simulink model "BugE_v0_40_MAS_loads_opt"  (R2015b)
settings: Solver=FixedStepDiscrete  StartTime=0.0  StopTime=1370  FixedStep=sample_time  RelTol=1e-3
values from neighbouring files (symbols this model uses):
  AB_diode_dV = 0.9    [main_sync.m]
  air_density = 1.225    [main_sync.m]
  bus_ac_Pmax_abs = 240    [main_sync.m]
  bus_charger_Pmax = 1000    [main_sync.m]
  bus_load_Pmax_abs = 260    [main_sync.m]
  capInitVolt = capVmax*sqrt(capInitSoC)    [main_sync.m]
  cyc_kph = [cyc_kph(:,1), cyc_kph(:,2)*speed_max_limit/speed_max]    [main_sync.m]
  cyc_repeat = 1    [main_sync.m]
  ess1_init_soc = 1    [main_sync.m]
  ess1_soh = 1    [main_sync.m]
  ess2_init_soc = 1    [main_sync.m]
  ess2_soh = 1    [main_sync.m]
  ess3_init_soc = 1    [main_sync.m]
  ess3_soh = 1    [main_sync.m]
  ess4_init_soc = 1    [main_sync.m]
  ess4_soh = 1    [main_sync.m]
  ess5_init_soc = 1    [main_sync.m]
  ess5_soh = 1    [main_sync.m]
  gear_ratio = 6    [main_sync.m]
  JADE_on = 0    [main_sync.m]
  loadpower = rawcsv(:,2)    [main_sync.m]
  loadtime = rawcsv(:,1)    [main_sync.m]
  lockSOCs = 0    [main_sync.m]
  max_brk_torque = 300    [main_sync.m]
  no_wheels = 3    [main_sync.m]
  perform_sample_time = 3*60    (= 180)    [main_sync.m]
  period2 = max(loadtime)    [main_sync.m]
  PV_Pmax = 100    [main_sync.m]
  sample_time = 0.01    [main_sync.m]
  startup_seq_step_delay = 0.2    [main_sync.m]
  stop_option = 0    [main_sync.m]
  use_drive_cycle = 1    [main_sync.m]
  use_real_subs_loads = 1    [main_sync.m]
  vbus_max = 25    [main_sync.m]
  vbus_min = 17    [main_sync.m]
  vbus_safety_threshold = 2    [main_sync.m]
  vbus_threshold = 20    [main_sync.m]
  veh_CD = 0.35    [main_sync.m]
  veh_FA = 1.543    [main_sync.m]
  veh_gravity = 9.81*veh_mass    (= 1863.9)    [main_sync.m]
  veh_mass = 190    [main_sync.m]
  wh_1st_rrc = 0.02    [main_sync.m]
  wh_bearing_frc = 0.0015    [main_sync.m]
  wh_inertia = 0.0556    [main_sync.m]
  wh_radius = 0.508/2    (= 0.254)    [main_sync.m]
undefined symbols (not defined in the file or in its folder): capC, capR, cyc_acc, cyc_avg_time_samples, cyc_brk, cyc_grade, cyc_key, DCM_eff_factor_for_Vin, DCM_eff_for_Iout, DCM_Iout, DCM_Iout_max, DCM_Pin_noload, DCM_Pout_max, DCM_Vin, DCM_Vout, DiscIntNeverNeededParam, ess2_coulombic_eff, ess2_Ineg_max_SOC, ess2_Ineg_max_temp, ess2_Ipos_max_SOC, ess2_Ipos_max_temp, ess2_max_ah_cap, ess2_max_volts, ess2_min_volts, ess2_module_parallel, ess2_module_series, ess2_r_dis, ess2_soc, ess2_SOC_for_Ilimit, ess2_temp_for_Ilimit, ess2_temp_max, ess2_tmp, ess2_voc, ess3_coulombic_eff, ess3_max_ah_cap, ess3_module_parallel, ess3_module_series, ess3_r_dis, ess3_soc, ess3_tmp, ess3_voc, ess_coulombic_eff, ess_Ineg_max_SOC, ess_Ineg_max_temp, ess_Ipos_max_SOC, ess_Ipos_max_temp, ess_max_ah_cap, ess_max_volts, ess_min_volts, ess_module_parallel, ess_module_series, ess_nominal_volts, ess_r_dis, ess_soc, ess_SOC_for_Ilimit, ess_temp_for_Ilimit, ess_temp_max, ess_tmp, ess_voc, MC_eff1 ... (+18)
libraries: simulink x142, dspstat3 x2, commfilt2 x1, simulink_extras x1
(part 5 of 7)

== system BugE_v0_40_MAS_loads_opt/Master Controller/DCDC Calculators/FE // CHG Class Voltage => Power Droop ==
  Vbus_min : Inport
  Vbus_max : Inport  Port=2
  Vbus : Inport  Port=3
  Pmax_spec : Inport  Port=4
  50ms moving avg : DiscreteFir  Coefficients=ones(1,0.05*(1/sample_time))/(0.05*(1/sample_time))  SampleTime=sample_time
  >=0 : Saturate  UpperLimit=inf  LowerLimit=0
  Constant6 : Constant  SampleTime=sample_time
  Divide : Product  Inputs=*/
  Product : Product
  Subtract1 : Sum  Inputs=+-
  Subtract2 : Sum  Inputs=++-
  Subtract3 : Sum  Inputs=+-
  Subtract4 : Sum  Inputs=+-
  Subtract5 : Sum  Inputs=-+
  "[0,1]" : Saturate  UpperLimit=1-eps  LowerLimit=0
  beta : Constant  Value=0.9  SampleTime=sample_time
  sqr : Math  Operator=square  SaturateOnIntegerOverflow=on
  vf : Product  Inputs=*/
  Pmax_lim : Outport
  wires:
  Product/1 -> >=0/1
  Divide/1 -> Subtract2/3
  beta/1 -> Subtract3/2
  Subtract3/1 -> sqr/1
  sqr/1 -> Subtract2/2, Divide/1
  Constant6/1 -> Subtract2/1, Subtract3/1, Subtract4/1
  vf/1 -> "[0,1]"/1
  Subtract4/1 -> Divide/2
  >=0/1 -> Pmax_lim/1
  Vbus/1 -> 50ms moving avg/1
  Vbus_min/1 -> Subtract5/1, Subtract1/2
  Vbus_max/1 -> Subtract5/2
  Subtract5/1 -> vf/2
  Subtract1/1 -> vf/1
  "[0,1]"/1 -> Subtract4/2
  Subtract2/1 -> Product/1
  Pmax_spec/1 -> Product/2
  50ms moving avg/1 -> Subtract1/1

== system BugE_v0_40_MAS_loads_opt/Master Controller/DCDC Calculators/LD Class Voltage => Power Droop ==
  Vbus_min : Inport
  Vbus_max : Inport  Port=2
  Vbus : Inport  Port=3
  Pmax_spec_abs : Inport  Port=4
  50ms moving avg : DiscreteFir  Commented=through  Coefficients=ones(1,0.05*(1/sample_time))/(0.05*(1/sample_time))  SampleTime=sample_time
  <=0 : Saturate  UpperLimit=0  LowerLimit=-inf
  Constant6 : Constant  SampleTime=sample_time
  Divide1 : Product  Inputs=*/
  Product : Product
  Scope : Scope  NumInputPorts=2
  Subtract : Sum  Inputs=--+
  Subtract1 : Sum  Inputs=+-
  Subtract2 : Sum  Inputs=+-
  Subtract5 : Sum  Inputs=-+
  "[0,1]" : Saturate  UpperLimit=1  LowerLimit=eps
  beta : Constant  Value=0.9  SampleTime=sample_time
  sqr : Math  Operator=square  SaturateOnIntegerOverflow=on
  vf : Product  Inputs=*/
  Pmax_lim (neg) : Outport
  wires:
  vf/1 -> Scope/1, "[0,1]"/1
  50ms moving avg/1 -> Subtract1/1
  Vbus_min/1 -> Subtract5/1, Subtract1/2
  Vbus_max/1 -> Subtract5/2
  Subtract5/1 -> vf/2
  Subtract1/1 -> vf/1
  Constant6/1 -> Subtract/1, Subtract2/1
  beta/1 -> Subtract2/2
  Divide1/1 -> Subtract/3
  Subtract2/1 -> sqr/1
  sqr/1 -> Subtract/2, Divide1/1
  "[0,1]"/1 -> Divide1/2
  <=0/1 -> Scope/2, Pmax_lim (neg)/1
  Subtract/1 -> Product/1
  Pmax_spec_abs/1 -> Product/2
  Product/1 -> <=0/1
  Vbus/1 -> 50ms moving avg/1

== system BugE_v0_40_MAS_loads_opt/Master Controller/DCDC Calculators/ones voltage cmd ==
  I : Inport
  2dbl : DataTypeConversion
  Bias : Bias  Bias=1
  Gain : Gain  Gain=0
  O : Outport
  wires:
  Gain/1 -> Bias/1
  I/1 -> 2dbl/1
  2dbl/1 -> Gain/1
  Bias/1 -> O/1

== system BugE_v0_40_MAS_loads_opt/Master Controller/DCDC Calculators/zeros power cmd ==
  I : Inport
  2dbl : DataTypeConversion
  Gain : Gain  Gain=0
  O : Outport
  wires:
  Gain/1 -> O/1
  I/1 -> 2dbl/1
  2dbl/1 -> Gain/1

== system BugE_v0_40_MAS_loads_opt/Master Controller/DCDC Calculators/zeros power cmd1 ==
  I : Inport
  2dbl : DataTypeConversion
  Gain : Gain  Gain=0
  O : Outport
  wires:
  Gain/1 -> O/1
  I/1 -> 2dbl/1
  2dbl/1 -> Gain/1

== system BugE_v0_40_MAS_loads_opt/Master Controller/Motor Controller/MB Class Current => Throttle Droop ==
  I : Inport
  Imax : Inport  Port=2
  Constant6 : Constant  SampleTime=sample_time
  Divide : Product  Inputs=*/
  If : Product  Inputs=*/
  Rate Limiter 0-full in 1s : RateLimiter  FallingSlewLimit=-1/sample_time  SampleTimeMode=inherited  LinearizeAsGain=off
  Subtract2 : Sum  Inputs=++-
  Subtract3 : Sum  Inputs=+-
  Subtract4 : Sum  Inputs=+-
  "[0, 1]" : Saturate  UpperLimit=1-eps  LowerLimit=0
  "[0,1-eps]" : Saturate  UpperLimit=1-eps  LowerLimit=0
  beta : Constant  Value=0.85  SampleTime=sample_time
  moving average 200ms : DiscreteFir  Coefficients=ones(1,20)/20  SampleTime=sample_time
  sqr : Math  Operator=square  SaturateOnIntegerOverflow=on
  thr_max_lim : Outport
  wires:
  Subtract2/1 -> "[0, 1]"/1
  Divide/1 -> Subtract2/3
  beta/1 -> Subtract3/2
  Subtract3/1 -> sqr/1
  sqr/1 -> Subtract2/2, Divide/1
  Constant6/1 -> Subtract2/1, Subtract3/1, Subtract4/1
  Subtract4/1 -> Divide/2
  "[0,1-eps]"/1 -> Subtract4/2
  Imax/1 -> If/2
  If/1 -> "[0,1-eps]"/1
  "[0, 1]"/1 -> Rate Limiter 0-full in 1s/1
  Rate Limiter 0-full in 1s/1 -> moving average 200ms/1
  moving average 200ms/1 -> thr_max_lim/1
  I/1 -> If/1

== system BugE_v0_40_MAS_loads_opt/Master Controller/Operating Mode Controller/Accessories (State 2) ==
  note: Disable for MB modules
      | where the DCDC is ok but
      | the battery is not usable;
      |
      | Enable for everything usable
  devices_ON bus : Inport
  Enable : EnablePort  StatesWhenEnabling=reset
  Bus Creator1 : BusCreator  Inputs=10
  Bus Creator2 : BusCreator  Inputs=5
  Bus Selector : BusSelector  OutputSignals=MBDCDC_on,MB_on,SBDCDC_on,SB_on,FEDCDC_on,FE_on,CHGDCDC_on,CHG_on,LDDCDC_on,LD_on
  Constant : Constant  OutDataTypeStr=boolean  SampleTime=sample_time
  and{5..9} (5 alike) : Logic  AllPortsSameDT=off  OutDataTypeStr=boolean
  not{,1..4} (5 alike) : Logic  Operator=NOT  AllPortsSameDT=off  OutDataTypeStr=boolean
  pass : Subsystem
  pass5 : Subsystem
  pass6 : Subsystem
  pass7 : Subsystem
  RLYs_and_12V bus : Outport  OutputWhenDisabled=reset  InitialOutput=0
  droop_bus : Outport  Port=2  OutputWhenDisabled=reset  InitialOutput=0
  wires:
  Constant/1 -> Bus Creator2/5  "RLY_DRV_DSBL"
  Bus Creator1/1 -> droop_bus/1
  devices_ON bus/1 -> Bus Selector/1
  and5/1 -> pass6/1(I), not/1, Bus Creator1/1  "MB_droop_EN"
  and7/1 -> not2/1, Bus Creator1/3  "FE_droop_EN"
  and8/1 -> not3/1, Bus Creator1/4  "CHG_droop_EN"
  and6/1 -> pass7/1(I), not1/1, Bus Creator1/2  "SB_droop_EN"
  and9/1 -> not4/1, Bus Creator1/5  "LD_droop_EN"
  Bus Selector/1 -> and5/1  "<MBDCDC_on>"
  Bus Selector/10 -> and9/2  "<LD_on>"
  Bus Selector/9 -> and9/1  "<LDDCDC_on>"
  Bus Selector/8 -> and8/2  "<CHG_on>"
  Bus Selector/7 -> and8/1  "<CHGDCDC_on>"
  Bus Selector/6 -> and7/2  "<FE_on>"
  Bus Selector/5 -> and7/1  "<FEDCDC_on>"
  Bus Selector/4 -> and6/2  "<SB_on>"
  Bus Selector/3 -> and6/1  "<SBDCDC_on>"
  Bus Selector/2 -> and5/2  "<MB_on>"
  not/1 -> pass5/1(I), Bus Creator1/6  "MB_droop_DSBL"
  not1/1 -> pass/1(I), Bus Creator1/7  "SB_droop_DSBL"
  not2/1 -> Bus Creator1/8  "FE_droop_DSBL"
  not3/1 -> Bus Creator1/9  "CHG_droop_DSBL"
  not4/1 -> Bus Creator1/10  "LD_droop_DSBL"
  Bus Creator2/1 -> RLYs_and_12V bus/1
  pass/1(O) -> Bus Creator2/1  "RLY_SB_DSBL"
  pass5/1(O) -> Bus Creator2/2  "RLY_MB_DSBL"
  pass6/1(O) -> Bus Creator2/3  "RLY_MB_EN"
  pass7/1(O) -> Bus Creator2/4  "RLY_SB_EN"

== system BugE_v0_40_MAS_loads_opt/Master Controller/Operating Mode Controller/Driving (State 3) ==
  note: Everything usable including
      | MB modules where the
      | DCDC is ok but the battery
      | is not usable (fail-mode)
  devices_ON bus : Inport
  Enable : EnablePort  StatesWhenEnabling=reset
  Bus Creator1 : BusCreator  Inputs=10
  Bus Creator2 : BusCreator  Inputs=5
  Bus Selector : BusSelector  OutputSignals=MBDCDC_on,MB_on,SBDCDC_on,SB_on,FEDCDC_on,FE_on,CHGDCDC_on,CHG_on,LDDCDC_on,LD_on
  Constant : Constant  OutDataTypeStr=boolean  SampleTime=sample_time
  and{6..9} (4 alike) : Logic  AllPortsSameDT=off  OutDataTypeStr=boolean
  not{,1..5} (6 alike) : Logic  Operator=NOT  AllPortsSameDT=off  OutDataTypeStr=boolean
  pass{2..5} (4 alike) : Logic  Operator=NOT  AllPortsSameDT=off  OutDataTypeStr=boolean
  through{2..5} (4 alike) : Logic  Operator=NOT  AllPortsSameDT=off  OutDataTypeStr=boolean
  RLYs_and_12V bus : Outport  OutputWhenDisabled=reset  InitialOutput=0
  droop_bus : Outport  Port=2  OutputWhenDisabled=reset  InitialOutput=0
  wires:
  Constant/1 -> Bus Creator2/5  "RLY_DRV_EN"
  Bus Creator1/1 -> droop_bus/1
  devices_ON bus/1 -> Bus Selector/1
  through5/1 -> Bus Creator1/1  "MB_droop_EN"
  and7/1 -> not2/1, Bus Creator1/3  "FE_droop_EN"
  and8/1 -> not3/1, Bus Creator1/4  "CHG_droop_EN"
  and6/1 -> pass4/1, not1/1, Bus Creator1/2  "SB_droop_EN"
  and9/1 -> not4/1, Bus Creator1/5  "LD_droop_EN"
  Bus Selector/1 -> not/1, pass5/1  "<MBDCDC_on>"
  Bus Selector/10 -> and9/2  "<LD_on>"
  Bus Selector/9 -> and9/1  "<LDDCDC_on>"
  Bus Selector/8 -> and8/2  "<CHG_on>"
  Bus Selector/7 -> and8/1  "<CHGDCDC_on>"
  Bus Selector/6 -> and7/2  "<FE_on>"
  Bus Selector/5 -> and7/1  "<FEDCDC_on>"
  Bus Selector/4 -> and6/2  "<SB_on>"
  Bus Selector/3 -> and6/1  "<SBDCDC_on>"
  Bus Selector/2 -> pass3/1, not5/1  "<MB_on>"
  not/1 -> Bus Creator1/6  "MB_droop_DSBL"
  not1/1 -> Bus Creator1/7, pass2/1  "SB_droop_DSBL"
  not2/1 -> Bus Creator1/8  "FE_droop_DSBL"
  not3/1 -> Bus Creator1/9  "CHG_droop_DSBL"
  not4/1 -> Bus Creator1/10  "LD_droop_DSBL"
  Bus Creator2/1 -> RLYs_and_12V bus/1
  pass2/1 -> through2/1
  through2/1 -> Bus Creator2/1  "RLY_SB_DSBL"
  not5/1 -> Bus Creator2/2  "RLY_MB_DSBL"
  pass3/1 -> through3/1
  through3/1 -> Bus Creator2/3  "RLY_MB_EN"
  pass4/1 -> through4/1
  through4/1 -> Bus Creator2/4  "RLY_SB_EN"
  pass5/1 -> through5/1

== system BugE_v0_40_MAS_loads_opt/Master Controller/Operating Mode Controller/Standby (State 0) ==
  devices_ON bus : Inport
  Enable : EnablePort  StatesWhenEnabling=reset
  Bus Creator : BusCreator  Inputs=5
  Bus Creator1 : BusCreator  Inputs=6
  Bus Creator2 : BusCreator  Inputs=5
  Bus Selector : BusSelector  OutputSignals=MBDCDC_on,SBDCDC_on,FEDCDC_on,CHGDCDC_on,LDDCDC_on
  dbl2bool{,1..15} (16 alike) : DataTypeConversion  OutDataTypeStr=boolean
  disable everything : Constant  OutDataTypeStr=double  SampleTime=sample_time
  ones : Subsystem
  ones1 : Subsystem
  ones2 : Subsystem
  ones3 : Subsystem
  ones4 : Subsystem
  RLYs_and_12V bus : Outport  OutputWhenDisabled=reset  InitialOutput=0
  module_PWR bus : Outport  Port=2  OutputWhenDisabled=reset  InitialOutput=0
  droop_bus : Outport  Port=3  OutputWhenDisabled=reset  InitialOutput=0
  wires:
  Bus Selector/1 -> ones/1(I)  "<MBDCDC_on>"
  Bus Selector/2 -> ones1/1(I)  "<SBDCDC_on>"
  Bus Selector/3 -> ones2/1(I)  "<FEDCDC_on>"
  Bus Selector/4 -> ones3/1(I)  "<CHGDCDC_on>"
  Bus Selector/5 -> ones4/1(I)  "<LDDCDC_on>"
  dbl2bool2/1 -> Bus Creator/1  "MB_droop_DSBL"
  dbl2bool1/1 -> Bus Creator/2  "SB_droop_DSBL"
  dbl2bool/1 -> Bus Creator/3  "FE_droop_DSBL"
  dbl2bool3/1 -> Bus Creator/5  "LD_droop_DSBL"
  dbl2bool4/1 -> Bus Creator/4  "CHG_droop_DSBL"
  Bus Creator/1 -> droop_bus/1
  devices_ON bus/1 -> Bus Selector/1  "detected and not turned off internally"
  Bus Creator2/1 -> module_PWR bus/1
  dbl2bool8/1 -> Bus Creator2/5  "LD_PWR_DSBL"
  dbl2bool9/1 -> Bus Creator2/4  "CHG_PWR_DSBL"
  dbl2bool5/1 -> Bus Creator2/3  "FE_PWR_DSBL"
  dbl2bool6/1 -> Bus Creator2/2  "SB_MOD_PWR_DSBL"
  dbl2bool7/1 -> Bus Creator2/1  "MB_MOD_PWR_DSBL"
  dbl2bool10/1 -> Bus Creator1/6  "RLY_SB_DSBL"
  dbl2bool11/1 -> Bus Creator1/5  "RLY_MB_DSBL"
  dbl2bool14/1 -> Bus Creator1/1  "DDC_DSBL"
  dbl2bool13/1 -> Bus Creator1/2  "RLY_EDLC_DSBL"
  dbl2bool12/1 -> Bus Creator1/3  "RLY_AUX_DSBL"
  dbl2bool15/1 -> Bus Creator1/4  "RLY_DRV_DSBL"
  disable everything/1 -> dbl2bool15/1, dbl2bool12/1, dbl2bool13/1, dbl2bool14/1
  Bus Creator1/1 -> RLYs_and_12V bus/1
  ones/1(O) -> dbl2bool7/1, dbl2bool10/1, dbl2bool2/1
  ones1/1(O) -> dbl2bool11/1, dbl2bool6/1, dbl2bool1/1
  ones2/1(O) -> dbl2bool5/1, dbl2bool/1
  ones3/1(O) -> dbl2bool9/1, dbl2bool4/1
  ones4/1(O) -> dbl2bool8/1, dbl2bool3/1

== system BugE_v0_40_MAS_loads_opt/Master Controller/Operating Mode Controller/Startup sequence (State 1) ==
  note: STEP 1.
      | 	enable module power
      | 	for All energy sources
      | STEP 2.
      | 	close EDLC relays (DOT)
      | STEP 3.
      | 	close BMU batt relays via CAN
      | STEP 4.
      | 	enable Droop control for
      | 	everything but loads
      |
      | When the bus is ready (charged)...
      |
      | STEP 5.
      | 	enable DDC, loads, Droop
      | 	for everything
      | STEP 6.
      | 	disable power for all modules
      | 	not being detected, and
      | 	set startup ready flag
  note: No loads or MB modules
      | where the DCDC is ok but
      | the battery is not usable
  note: No MB modules where
      | the DCDC is ok but
      | the battery is not usable
  devices_ON bus : Inport
  bus ready : Inport  Port=2
  Enable : EnablePort  StatesWhenEnabling=reset
  Bus Creator1 : BusCreator  Inputs=5
  Bus Creator2 : BusCreator  Inputs=10
  Bus Selector2 : BusSelector  OutputSignals=LDDCDC_on,MBDCDC_on,SBDCDC_on,FEDCDC_on,CHGDCDC_on,MB_on,SB_on,FE_on,CHG_on,LD_on
  Switch : Switch  Criteria=u2 > Threshold
  Switch1 : Switch  Criteria=u2 > Threshold
  and{,1..11} (12 alike) : Logic  AllPortsSameDT=off  OutDataTypeStr=boolean
  choose_droop_activations : Subsystem  TreatAsAtomicUnit=on
  choose_droop_activations1 : Subsystem  TreatAsAtomicUnit=on
  nor{,1..4} (5 alike) : Logic  Operator=NOR  AllPortsSameDT=off  OutDataTypeStr=boolean
  ones : Subsystem
  ones1 : Subsystem
  ones2 : Subsystem
  ones3 : Subsystem
  ones4 : Subsystem
  pass : Subsystem
  pass1 : Subsystem
  start : Constant  OutDataTypeStr=boolean  SampleTime=sample_time
  startup_seq_step_delay w/ latch : Subsystem
  zeros : Subsystem
  RLYs_and_12V bus : Outport  OutputWhenDisabled=reset  InitialOutput=0
  droop_bus : Outport  Port=2  OutputWhenDisabled=reset  InitialOutput=0
  SUR : Outport  Port=3  OutputWhenDisabled=reset  InitialOutput=0
  module_PWR bus : Outport  Port=4  OutputWhenDisabled=reset  InitialOutput=0
  wires:
  startup_seq_step_delay w/ latch/2(delayed 2x) -> and2/1, and/1
  startup_seq_step_delay w/ latch/3(delayed 3x) -> Switch1/2, choose_droop_activations/Enable
  bus ready/1 -> startup_seq_step_delay w/ latch/2(bus ready)
  Switch/1 -> droop_bus/1
  choose_droop_activations1/1(droop_EN bus) -> Switch/1
  and1/1 -> Bus Creator2/6  "MB_MOD_PWR_EN"
  and4/1 -> Bus Creator2/7  "SB_MOD_PWR_EN"
  ones1/1(O) -> and3/1
  Switch1/1 -> Switch/3
  and5/1 -> Bus Creator2/10  "LD_PWR_EN"
  and6/1 -> Bus Creator2/9  "CHG_PWR_EN"
  and3/1 -> Bus Creator2/8  "FE_PWR_EN"
  and2/1 -> Bus Creator1/3  "RLY_SB_EN"
  and/1 -> Bus Creator1/2  "RLY_MB_EN"
  pass/1(O) -> Bus Creator1/4  "DDC_EN"
  pass1/1(O) -> Bus Creator1/5  "RLY_AUX_EN"
  Bus Creator1/1 -> RLYs_and_12V bus/1
  start/1 -> and6/2, and1/2, and4/2, and3/2, startup_seq_step_delay w/ latch/1(sigin)
  ones2/1(O) -> and4/1
  ones3/1(O) -> and6/1
  Bus Selector2/7 -> nor1/2, ones2/1(I)  "<SB_on>"
  Bus Selector2/9 -> nor3/2, ones3/1(I)  "<CHG_on>"
  startup_seq_step_delay w/ latch/1(delayed) -> Bus Creator1/1  "RLY_EDLC_EN"
  Bus Selector2/8 -> nor2/2, ones1/1(I), and2/2  "<FE_on>"
  Bus Selector2/6 -> ones/1(I), nor/2, and/2  "<MB_on>"
  ones/1(O) -> and1/1
  startup_seq_step_delay w/ latch/4(delayed 4x & BR) -> and5/2, choose_droop_activations1/Enable, Switch/2, pass1/1(I), pass/1(I)
  choose_droop_activations/1(droop_EN bus) -> Switch1/1
  zeros/1(O) -> Switch1/3
  devices_ON bus/1 -> choose_droop_activations/1(devices_ON bus), choose_droop_activations1/1(devices_ON bus), zeros/1(I), Bus Selector2/1
  Bus Selector2/2 -> nor/1  "<MBDCDC_on>"
  Bus Selector2/10 -> nor4/2, ones4/1(I)  "<LD_on>"
  Bus Selector2/1 -> nor4/1  "<LDDCDC_on>"
  Bus Selector2/5 -> nor3/1  "<CHGDCDC_on>"
  Bus Selector2/4 -> nor2/1  "<FEDCDC_on>"
  Bus Selector2/3 -> nor1/1  "<SBDCDC_on>"
  and7/1 -> Bus Creator2/2  "MB_PWR_DSBL"
  and8/1 -> Bus Creator2/3  "SB_PWR_DSBL"
  and9/1 -> Bus Creator2/4  "FE_PWR_DSBL"
  and10/1 -> Bus Creator2/5  "CHG_PWR_DSBL"
  and11/1 -> Bus Creator2/1  "LD_PWR_DSBL"
  Bus Creator2/1 -> module_PWR bus/1
  nor2/1 -> and9/2
  nor1/1 -> and8/2
  nor/1 -> and7/2
  nor3/1 -> and10/2
  nor4/1 -> and11/1
  startup_seq_step_delay w/ latch/5((d4x & BR) delayed 2x) -> and10/1, and9/1, and8/1, and7/1, and11/2, SUR/1
  ones4/1(O) -> and5/1

== system BugE_v0_40_MAS_loads_opt/Master Controller/Operating Mode Controller/State machine 0 std, 1 startup, 2 acc, 3 drv, 4 fault ==
  ACC : Inport
  IGON : Inport  Port=2
  RFD (ready for driving) : Inport  Port=3
  SUR (startup ready) : Inport  Port=4
  ESTOP (user triggered e-stop) : Inport  Port=5
  0 => 1 : Subsystem  TreatAsAtomicUnit=on
  1 => 2 : Subsystem  TreatAsAtomicUnit=on
  2 => 3 : Subsystem  TreatAsAtomicUnit=on
  3 => 2 : Subsystem  TreatAsAtomicUnit=on
  ==0 : simulink/Logic and Bit Operations/Compare To Constant  relop===  const=0  OutDataTypeStr=boolean
  ==1 : simulink/Logic and Bit Operations/Compare To Constant  relop===  const=1  OutDataTypeStr=boolean
  ==2 : simulink/Logic and Bit Operations/Compare To Constant  relop===  const=2  OutDataTypeStr=boolean
  ==3 : simulink/Logic and Bit Operations/Compare To Constant  relop===  const=3  OutDataTypeStr=boolean
  All => 0 : Subsystem  TreatAsAtomicUnit=on
  If : If  NumInputs=6  IfExpression=((~u2) & (~u3)) | u6  ElseIfExpressions="(u1==0) & u2,  (u1==1) & u2 & u4,  (u1==2) & u3 & u5,  (u1==3) & ((~u3)|(~u5))"
  New state Default 0 : Merge  Inputs=6  InitialOutput=0
  Old state 1 : UnitDelay  SampleTime=sample_time
  bool2dbl {2..6} (5 alike) : DataTypeConversion  OutDataTypeStr=double
  maintain : Subsystem  TreatAsAtomicUnit=on
  pass10 : Subsystem
  pass2 : Subsystem
  pass3 : Subsystem
  pass4 : Subsystem
  pass5 : Subsystem
  state : Outport
  enable_standby : Outport  Port=2
  enable_startup : Outport  Port=3
  enable_accessories : Outport  Port=4
  enable_driving : Outport  Port=5
  wires:
  pass5/1(O) -> bool2dbl 5/1  "ems_SM_RFD"
  If/1 -> All => 0/Action
  If/2 -> 0 => 1/Action
  If/3 -> 1 => 2/Action
  If/4 -> 2 => 3/Action
  If/5 -> 3 => 2/Action
  If/6 -> maintain/Action
  3 => 2/1(new) -> New state Default 0/5
  maintain/1(new) -> New state Default 0/6
  pass2/1(O) -> bool2dbl 2/1  "ems_SM_ACC"
  pass3/1(O) -> bool2dbl 3/1  "ems_SM_IGON"
  ==1/1 -> enable_startup/1
  ==2/1 -> enable_accessories/1
  ==3/1 -> enable_driving/1
  ==0/1 -> enable_standby/1
  pass4/1(O) -> bool2dbl 4/1  "ems_SM_SUR"
  bool2dbl 3/1 -> If/3
  bool2dbl 2/1 -> If/2
  bool2dbl 5/1 -> If/5
  bool2dbl 4/1 -> If/4
  bool2dbl 6/1 -> If/6
  New state Default 0/1 -> ==3/1, ==2/1, ==1/1, Old state 1/1, state/1, ==0/1  "ems_SM_state"
  Old state 1/1 -> If/1, maintain/1(prev)
  All => 0/1(new) -> New state Default 0/1
  2 => 3/1(new) -> New state Default 0/4
  1 => 2/1(new) -> New state Default 0/3
  0 => 1/1(new) -> New state Default 0/2
  pass10/1(O) -> bool2dbl 6/1  "ems_SM_ESTOP"
  ACC/1 -> pass2/1(I)
  IGON/1 -> pass3/1(I)
  SUR (startup ready)/1 -> pass4/1(I)
  RFD (ready for driving)/1 -> pass5/1(I)
  ESTOP (user triggered e-stop)/1 -> pass10/1(I)

== system BugE_v0_40_MAS_loads_opt/Master Controller/Operating Mode Controller/bus charged & within limits ==
  < vbus_max + (...) : RelationalOperator  Operator=<  OutDataTypeStr=boolean
  >= vbus_threshold : simulink/Logic and Bit Operations/Compare To Constant  relop=>=  const=vbus_threshold  OutDataTypeStr=boolean
  Add : Sum
  Logical Operator : Logic  AllPortsSameDT=off  OutDataTypeStr=boolean
  vbus_max : Constant  Value=vbus_max  SampleTime=sample_time
  vbus_safety_threshold : Constant  Value=vbus_safety_threshold  SampleTime=sample_time
  bus_ready : Outport
  wires:
  >= vbus_threshold/1 -> Logical Operator/1
  [Vcap_reading] -> < vbus_max + (...)/1, >= vbus_threshold/1
  Add/1 -> < vbus_max + (...)/2
  vbus_max/1 -> Add/1
  vbus_safety_threshold/1 -> Add/2
  Logical Operator/1 -> bus_ready/1
  < vbus_max + (...)/1 -> Logical Operator/2

== system BugE_v0_40_MAS_loads_opt/Master Controller/Operating Mode Controller/ready for driving ==
  Bus Selector : BusSelector  OutputSignals=MBDCDC_on,MB_on
  From11 : From  Commented=on  GotoTag=CHGDCDC_detected  TagVisibility=global
  From12 : From  Commented=on  GotoTag=CHG_detected  TagVisibility=global
  a charger connected : Logic  Operator=OR  Inputs=1  AllPortsSameDT=off  OutDataTypeStr=boolean
  able to power motor : Logic  Inputs=1  AllPortsSameDT=off  OutDataTypeStr=boolean
  and : Logic  AllPortsSameDT=off  OutDataTypeStr=boolean
  no charger connected : Logic  Operator=NOT  Inputs=1  AllPortsSameDT=off  OutDataTypeStr=boolean
  or : Logic  Operator=OR  AllPortsSameDT=off  OutDataTypeStr=boolean
  ready : Logic  AllPortsSameDT=off  OutDataTypeStr=boolean
  RFD : Outport
  wires:
  and/1 -> a charger connected/1
  ready/1 -> RFD/1
  or/1 -> able to power motor/1
  no charger connected/1 -> ready/1
  able to power motor/1 -> ready/2
  From12/1 -> and/2
  From11/1 -> and/1
  [devices_ON_bus] -> Bus Selector/1
  Bus Selector/1 -> or/1  "<MBDCDC_on>"
  Bus Selector/2 -> or/2  "<MB_on>"
  a charger connected/1 -> no charger connected/1

== system BugE_v0_40_MAS_loads_opt/Master Controller/Operating Mode Controller/start-up ready ==
  Compare To Zero : simulink/Logic and Bit Operations/Compare To Zero  relop===  OutDataTypeStr=boolean
  S-R Flip-Flop : simulink_extras/Flip Flops/S-R Flip-Flop  initial_condition=0
  Terminator : Terminator
  Unit Delay : UnitDelay  SampleTime=sample_time
  Unit Delay1 : UnitDelay  SampleTime=sample_time
  SUR : Outport
  wires:
  [SM_SUR_flag] -> Unit Delay/1
  [state] -> Unit Delay1/1
  Unit Delay/1 -> S-R Flip-Flop/1
  Compare To Zero/1 -> S-R Flip-Flop/2
  Unit Delay1/1 -> Compare To Zero/1
  S-R Flip-Flop/1 -> SUR/1
  S-R Flip-Flop/2 -> Terminator/1

== system BugE_v0_40_MAS_loads_opt/Master Controller/Secondary Objectives/MB SOC balancing ==
  enable : Inport
  "Balancing type: 1: none, 2: P>0, 3: P<0" : Subsystem
  Bus Selector : BusSelector  OutputSignals=MB_droop
  MB balancing through load distribution : Subsystem
  Mux1 : Mux  Inputs=2
  Mux2 : Mux  Inputs=2
  Scope : Scope
  and : Logic  AllPortsSameDT=off  OutDataTypeStr=boolean
  MB slope adj : Outport
  wires:
  MB balancing through load distribution/1(MB slope adj) -> MB slope adj/1
  enable/1 -> "Balancing type: 1: none, 2: P>0, 3: P<0"/1(enable)
  Mux1/1 -> "Balancing type: 1: none, 2: P>0, 3: P<0"/2(DCDC Iout (bus side))
  [active_droop_bus] -> Bus Selector/1
  [RLY_MB] -> and/2
  "Balancing type: 1: none, 2: P>0, 3: P<0"/1(type) -> MB balancing through load distribution/1(distribution type), Scope/1
  Mux2/1 -> MB balancing through load distribution/3(MB SOCs)
  and/1 -> "Balancing type: 1: none, 2: P>0, 3: P<0"/3(enabled MODs), MB balancing through load distribution/2(MOD's EN)
  Bus Selector/1 -> and/1  "<MB_droop>"
  [Iout_MB1_DCDC_reading] -> Mux1/1
  [Iout_MB2_DCDC_reading] -> Mux1/2
  [SOC_MB1_received] -> Mux2/1
  [SOC_MB2_received] -> Mux2/2

== system BugE_v0_40_MAS_loads_opt/Master Controller/Secondary Objectives/Motor MBDCDC boost ==
  enable : Inport
  Bus Selector : BusSelector  OutputSignals=MB_droop
  Product : Product
  Saturation : Saturate  UpperLimit=0  LowerLimit=vbus_min-vbus_max
  Switch1 : Switch  Criteria=u2 > Threshold
  "[0.05, inf)" : DeadZone  LowerValue=-inf  UpperValue=0.05  SaturateOnIntegerOverflow=on
  boost off : Logic  Operator=NOT  AllPortsSameDT=off  OutDataTypeStr=boolean
  d Imotor / d t : simulink/Discrete/Discrete Derivative  gainval=1.0  ICPrevScaledInput=0.0  InputProcessing=Inherited  OutMin=[]  OutMax=[]  OutDataType=fixdt(1, 16)  OutScaling=2^-10  DoSatur=off
  moving average 50ms : DiscreteFir  Coefficients=ones(1,5)/5  SampleTime=sample_time
  normalize 1 / Imax : Gain  Gain=1/mc_max_crrnt
  ones : Subsystem
  shift gain [d_V0/ (d_I/d_t)] : Gain  Gain=-25
  some MB DCDCs are off : Logic  Operator=NAND  Inputs=1  AllPortsSameDT=off  OutDataTypeStr=boolean
  use boost : Logic  Operator=NOR  AllPortsSameDT=off  OutDataTypeStr=boolean
  zero : Constant  Value=0  SampleTime=sample_time
  MB V0 adj : Outport
  wires:
  shift gain [d_V0/ (d_I/d_t)]/1 -> Saturation/1
  moving average 50ms/1 -> normalize 1 / Imax/1
  enable/1 -> boost off/1
  boost off/1 -> use boost/2
  use boost/1 -> Switch1/2
  some MB DCDCs are off/1 -> use boost/1
  Product/1 -> Switch1/1
  zero/1 -> Switch1/3
  ones/1(O) -> Product/2
  normalize 1 / Imax/1 -> d Imotor / d t/1
  [Drive_current_reading] -> moving average 50ms/1
  Switch1/1 -> MB V0 adj/1
  d Imotor / d t/1 -> "[0.05, inf)"/1
  "[0.05, inf)"/1 -> shift gain [d_V0/ (d_I/d_t)]/1
  Saturation/1 -> Product/1
  [active_droop_bus] -> Bus Selector/1
  Bus Selector/1 -> ones/1(I), some MB DCDCs are off/1  "<MB_droop>"

== system BugE_v0_40_MAS_loads_opt/Master Controller/Secondary Objectives/Source prioritization ==
  enable : Inport
  Bias : Bias  Bias=1
  Bus Selector1 : BusSelector  OutputSignals=CHG_droop,MB_droop,SB_droop
  Gain : Gain  Gain=-1
  Gain1 : Gain  Gain=-2
  Product : Product
  Product1 : Product
  and1 : Logic  AllPortsSameDT=off  OutDataTypeStr=boolean
  and2 : Logic  AllPortsSameDT=off  OutDataTypeStr=boolean
  bool2dbl : DataTypeConversion  OutDataTypeStr=double
  bool2dbl1 : DataTypeConversion  OutDataTypeStr=double
  bool2dbl2 : DataTypeConversion  OutDataTypeStr=double
  charging : Logic  Operator=OR  Inputs=1  AllPortsSameDT=off  OutDataTypeStr=boolean
  SB slope adj : Outport
  MB V0 adj : Outport  Port=2
  SB V0 adj : Outport  Port=3
  wires:
  Bus Selector1/3 -> and1/1  "<SB_droop>"
  Bus Selector1/1 -> charging/1  "<CHG_droop>"
  charging/1 -> bool2dbl/1
  [active_droop_bus] -> Bus Selector1/1
  bool2dbl/1 -> Product1/1, Product/1
  Product/1 -> Gain1/1
  Product1/1 -> Gain/1
  Bias/1 -> SB slope adj/1
  and2/1 -> bool2dbl1/1
  bool2dbl2/1 -> Bias/1, Product1/2
  bool2dbl1/1 -> Product/2
  enable/1 -> and2/2, and1/2
  and1/1 -> bool2dbl2/1
  Bus Selector1/2 -> and2/1  "<MB_droop>"
  Gain1/1 -> MB V0 adj/1
  Gain/1 -> SB V0 adj/1

== system BugE_v0_40_MAS_loads_opt/Master Controller/Signal Buffer/(0 device OFF // 1 ON)1 ==
  EN : Inport
  DSBL : Inport  Port=2
  2dbl : DataTypeConversion  OutDataTypeStr=double
  2dbl1 : DataTypeConversion  OutDataTypeStr=double
  Detect Increase : simulink/Logic and Bit Operations/Detect Increase  vinit=0.0  InputProcessing=Inherited  OutDataTypeStr=boolean
  Detect Increase1 : simulink/Logic and Bit Operations/Detect Increase  vinit=0.0  InputProcessing=Inherited  OutDataTypeStr=boolean
  OR : Sum
  Switch : Switch  Criteria=u2 > Threshold
  Switch1 : Switch  Criteria=u2 > Threshold
  Unit Delay : UnitDelay  SampleTime=sample_time
  disable : Constant  Value=0  OutDataTypeStr=boolean  SampleTime=sample_time
  enable : Constant  OutDataTypeStr=boolean  SampleTime=sample_time
  state : Outport
  wires:
  EN/1 -> Detect Increase/1
  Detect Increase1/1 -> 2dbl1/1
  Switch/1 -> state/1, Unit Delay/1
  DSBL/1 -> Detect Increase1/1
  OR/1 -> Switch/2
  Detect Increase/1 -> 2dbl/1
  Unit Delay/1 -> Switch/3
  disable/1 -> Switch1/1
  enable/1 -> Switch1/3
  Switch1/1 -> Switch/1
  2dbl1/1 -> Switch1/2, OR/2
  2dbl/1 -> OR/1

== system BugE_v0_40_MAS_loads_opt/Master Controller/Signal Buffer/(0 device OFF // 1 ON)10 ==
  EN : Inport
  DSBL : Inport  Port=2
  2dbl : DataTypeConversion  OutDataTypeStr=double
  2dbl1 : DataTypeConversion  OutDataTypeStr=double
  Detect Increase : simulink/Logic and Bit Operations/Detect Increase  vinit=0.0  InputProcessing=Inherited  OutDataTypeStr=boolean
  Detect Increase1 : simulink/Logic and Bit Operations/Detect Increase  vinit=0.0  InputProcessing=Inherited  OutDataTypeStr=boolean
  OR : Sum
  Switch : Switch  Criteria=u2 > Threshold
  Switch1 : Switch  Criteria=u2 > Threshold
  Unit Delay : UnitDelay  SampleTime=sample_time
  disable : Constant  Value=0  OutDataTypeStr=boolean  SampleTime=sample_time
  enable : Constant  OutDataTypeStr=boolean  SampleTime=sample_time
  state : Outport
  wires:
  EN/1 -> Detect Increase/1
  Detect Increase1/1 -> 2dbl1/1
  Switch/1 -> state/1, Unit Delay/1
  DSBL/1 -> Detect Increase1/1
  OR/1 -> Switch/2
  Detect Increase/1 -> 2dbl/1
  Unit Delay/1 -> Switch/3
  disable/1 -> Switch1/1
  enable/1 -> Switch1/3
  Switch1/1 -> Switch/1
  2dbl1/1 -> Switch1/2, OR/2
  2dbl/1 -> OR/1

== system BugE_v0_40_MAS_loads_opt/Master Controller/Signal Buffer/(0 device OFF // 1 ON)11 ==
  EN : Inport
  DSBL : Inport  Port=2
  2dbl : DataTypeConversion  OutDataTypeStr=double
  2dbl1 : DataTypeConversion  OutDataTypeStr=double
  Detect Increase : simulink/Logic and Bit Operations/Detect Increase  vinit=0.0  InputProcessing=Inherited  OutDataTypeStr=boolean
  Detect Increase1 : simulink/Logic and Bit Operations/Detect Increase  vinit=0.0  InputProcessing=Inherited  OutDataTypeStr=boolean
  OR : Sum
  Switch : Switch  Criteria=u2 > Threshold
  Switch1 : Switch  Criteria=u2 > Threshold
  Unit Delay : UnitDelay  SampleTime=sample_time
  disable : Constant  Value=0  OutDataTypeStr=boolean  SampleTime=sample_time
  enable : Constant  OutDataTypeStr=boolean  SampleTime=sample_time
  state : Outport
  wires:
  EN/1 -> Detect Increase/1
  Detect Increase1/1 -> 2dbl1/1
  Switch/1 -> state/1, Unit Delay/1
  DSBL/1 -> Detect Increase1/1
  OR/1 -> Switch/2
  Detect Increase/1 -> 2dbl/1
  Unit Delay/1 -> Switch/3
  disable/1 -> Switch1/1
  enable/1 -> Switch1/3
  Switch1/1 -> Switch/1
  2dbl1/1 -> Switch1/2, OR/2
  2dbl/1 -> OR/1

== system BugE_v0_40_MAS_loads_opt/Master Controller/Signal Buffer/(0 device OFF // 1 ON)12 ==
  EN : Inport
  DSBL : Inport  Port=2
  2dbl : DataTypeConversion  OutDataTypeStr=double
  2dbl1 : DataTypeConversion  OutDataTypeStr=double
  Detect Increase : simulink/Logic and Bit Operations/Detect Increase  vinit=0.0  InputProcessing=Inherited  OutDataTypeStr=boolean
  Detect Increase1 : simulink/Logic and Bit Operations/Detect Increase  vinit=0.0  InputProcessing=Inherited  OutDataTypeStr=boolean
  OR : Sum
  Switch : Switch  Criteria=u2 > Threshold
  Switch1 : Switch  Criteria=u2 > Threshold
  Unit Delay : UnitDelay  SampleTime=sample_time
  disable : Constant  Value=0  OutDataTypeStr=boolean  SampleTime=sample_time
  enable : Constant  OutDataTypeStr=boolean  SampleTime=sample_time
  state : Outport
  wires:
  EN/1 -> Detect Increase/1
  Detect Increase1/1 -> 2dbl1/1
  Switch/1 -> state/1, Unit Delay/1
  DSBL/1 -> Detect Increase1/1
  OR/1 -> Switch/2
  Detect Increase/1 -> 2dbl/1
  Unit Delay/1 -> Switch/3
  disable/1 -> Switch1/1
  enable/1 -> Switch1/3
  Switch1/1 -> Switch/1
  2dbl1/1 -> Switch1/2, OR/2
  2dbl/1 -> OR/1

== system BugE_v0_40_MAS_loads_opt/Master Controller/Signal Buffer/(0 device OFF // 1 ON)13 ==
  EN : Inport
  DSBL : Inport  Port=2
  2dbl : DataTypeConversion  OutDataTypeStr=double
  2dbl1 : DataTypeConversion  OutDataTypeStr=double
  Detect Increase : simulink/Logic and Bit Operations/Detect Increase  vinit=0.0  InputProcessing=Inherited  OutDataTypeStr=boolean
  Detect Increase1 : simulink/Logic and Bit Operations/Detect Increase  vinit=0.0  InputProcessing=Inherited  OutDataTypeStr=boolean
  OR : Sum
  Switch : Switch  Criteria=u2 > Threshold
  Switch1 : Switch  Criteria=u2 > Threshold
  Unit Delay : UnitDelay  SampleTime=sample_time
  disable : Constant  Value=0  OutDataTypeStr=boolean  SampleTime=sample_time
  enable : Constant  OutDataTypeStr=boolean  SampleTime=sample_time
  state : Outport
  wires:
  EN/1 -> Detect Increase/1
  Detect Increase1/1 -> 2dbl1/1
  Switch/1 -> state/1, Unit Delay/1
  DSBL/1 -> Detect Increase1/1
  OR/1 -> Switch/2
  Detect Increase/1 -> 2dbl/1
  Unit Delay/1 -> Switch/3
  disable/1 -> Switch1/1
  enable/1 -> Switch1/3
  Switch1/1 -> Switch/1
  2dbl1/1 -> Switch1/2, OR/2
  2dbl/1 -> OR/1

== system BugE_v0_40_MAS_loads_opt/Master Controller/Signal Buffer/(0 device OFF // 1 ON)14 ==
  EN : Inport
  DSBL : Inport  Port=2
  2dbl : DataTypeConversion  OutDataTypeStr=double
  2dbl1 : DataTypeConversion  OutDataTypeStr=double
  Detect Increase : simulink/Logic and Bit Operations/Detect Increase  vinit=0.0  InputProcessing=Inherited  OutDataTypeStr=boolean
  Detect Increase1 : simulink/Logic and Bit Operations/Detect Increase  vinit=0.0  InputProcessing=Inherited  OutDataTypeStr=boolean
  OR : Sum
  Switch : Switch  Criteria=u2 > Threshold
  Switch1 : Switch  Criteria=u2 > Threshold
  Unit Delay : UnitDelay  SampleTime=sample_time
  disable : Constant  Value=0  OutDataTypeStr=boolean  SampleTime=sample_time
  enable : Constant  OutDataTypeStr=boolean  SampleTime=sample_time
  state : Outport
  wires:
  EN/1 -> Detect Increase/1
  Detect Increase1/1 -> 2dbl1/1
  Switch/1 -> state/1, Unit Delay/1
  DSBL/1 -> Detect Increase1/1
  OR/1 -> Switch/2
  Detect Increase/1 -> 2dbl/1
  Unit Delay/1 -> Switch/3
  disable/1 -> Switch1/1
  enable/1 -> Switch1/3
  Switch1/1 -> Switch/1
  2dbl1/1 -> Switch1/2, OR/2
  2dbl/1 -> OR/1

== system BugE_v0_40_MAS_loads_opt/Master Controller/Signal Buffer/(0 device OFF // 1 ON)15 ==
  EN : Inport
  DSBL : Inport  Port=2
  2dbl : DataTypeConversion  OutDataTypeStr=double
  2dbl1 : DataTypeConversion  OutDataTypeStr=double
  Detect Increase : simulink/Logic and Bit Operations/Detect Increase  vinit=0.0  InputProcessing=Inherited  OutDataTypeStr=boolean
  Detect Increase1 : simulink/Logic and Bit Operations/Detect Increase  vinit=0.0  InputProcessing=Inherited  OutDataTypeStr=boolean
  OR : Sum
  Switch : Switch  Criteria=u2 > Threshold
  Switch1 : Switch  Criteria=u2 > Threshold
  Unit Delay : UnitDelay  SampleTime=sample_time
  disable : Constant  Value=0  OutDataTypeStr=boolean  SampleTime=sample_time
  enable : Constant  OutDataTypeStr=boolean  SampleTime=sample_time
  state : Outport
  wires:
  EN/1 -> Detect Increase/1
  Detect Increase1/1 -> 2dbl1/1
  Switch/1 -> state/1, Unit Delay/1
  DSBL/1 -> Detect Increase1/1
  OR/1 -> Switch/2
  Detect Increase/1 -> 2dbl/1
  Unit Delay/1 -> Switch/3
  disable/1 -> Switch1/1
  enable/1 -> Switch1/3
  Switch1/1 -> Switch/1
  2dbl1/1 -> Switch1/2, OR/2
  2dbl/1 -> OR/1

== system BugE_v0_40_MAS_loads_opt/Master Controller/Signal Buffer/(0 device OFF // 1 ON)16 ==
  EN : Inport
  DSBL : Inport  Port=2
  2dbl : DataTypeConversion  OutDataTypeStr=double
  2dbl1 : DataTypeConversion  OutDataTypeStr=double
  Detect Increase : simulink/Logic and Bit Operations/Detect Increase  vinit=0.0  InputProcessing=Inherited  OutDataTypeStr=boolean
  Detect Increase1 : simulink/Logic and Bit Operations/Detect Increase  vinit=0.0  InputProcessing=Inherited  OutDataTypeStr=boolean
  OR : Sum
  Switch : Switch  Criteria=u2 > Threshold
  Switch1 : Switch  Criteria=u2 > Threshold
  Unit Delay : UnitDelay  SampleTime=sample_time
  disable : Constant  Value=0  OutDataTypeStr=boolean  SampleTime=sample_time
  enable : Constant  OutDataTypeStr=boolean  SampleTime=sample_time
  state : Outport
  wires:
  EN/1 -> Detect Increase/1
  Detect Increase1/1 -> 2dbl1/1
  Switch/1 -> state/1, Unit Delay/1
  DSBL/1 -> Detect Increase1/1
  OR/1 -> Switch/2
  Detect Increase/1 -> 2dbl/1
  Unit Delay/1 -> Switch/3
  disable/1 -> Switch1/1
  enable/1 -> Switch1/3
  Switch1/1 -> Switch/1
  2dbl1/1 -> Switch1/2, OR/2
  2dbl/1 -> OR/1

== system BugE_v0_40_MAS_loads_opt/Master Controller/Signal Buffer/(0 device OFF // 1 ON)2 ==
  EN : Inport
  DSBL : Inport  Port=2
  2dbl : DataTypeConversion  OutDataTypeStr=double
  2dbl1 : DataTypeConversion  OutDataTypeStr=double
  Detect Increase : simulink/Logic and Bit Operations/Detect Increase  vinit=0.0  InputProcessing=Inherited  OutDataTypeStr=boolean
  Detect Increase1 : simulink/Logic and Bit Operations/Detect Increase  vinit=0.0  InputProcessing=Inherited  OutDataTypeStr=boolean
  OR : Sum
  Switch : Switch  Criteria=u2 > Threshold
  Switch1 : Switch  Criteria=u2 > Threshold
  Unit Delay : UnitDelay  SampleTime=sample_time
  disable : Constant  Value=0  OutDataTypeStr=boolean  SampleTime=sample_time
  enable : Constant  OutDataTypeStr=boolean  SampleTime=sample_time
  state : Outport
  wires:
  EN/1 -> Detect Increase/1
  Detect Increase1/1 -> 2dbl1/1
  Switch/1 -> state/1, Unit Delay/1
  DSBL/1 -> Detect Increase1/1
  OR/1 -> Switch/2
  Detect Increase/1 -> 2dbl/1
  Unit Delay/1 -> Switch/3
  disable/1 -> Switch1/1
  enable/1 -> Switch1/3
  Switch1/1 -> Switch/1
  2dbl1/1 -> Switch1/2, OR/2
  2dbl/1 -> OR/1

== system BugE_v0_40_MAS_loads_opt/Master Controller/Signal Buffer/(0 device OFF // 1 ON)3 ==
  EN : Inport
  DSBL : Inport  Port=2
  2dbl : DataTypeConversion  OutDataTypeStr=double
  2dbl1 : DataTypeConversion  OutDataTypeStr=double
  Detect Increase : simulink/Logic and Bit Operations/Detect Increase  vinit=0.0  InputProcessing=Inherited  OutDataTypeStr=boolean
  Detect Increase1 : simulink/Logic and Bit Operations/Detect Increase  vinit=0.0  InputProcessing=Inherited  OutDataTypeStr=boolean
  OR : Sum
  Switch : Switch  Criteria=u2 > Threshold
  Switch1 : Switch  Criteria=u2 > Threshold
  Unit Delay : UnitDelay  SampleTime=sample_time
  disable : Constant  Value=0  OutDataTypeStr=boolean  SampleTime=sample_time
  enable : Constant  OutDataTypeStr=boolean  SampleTime=sample_time
  state : Outport
  wires:
  EN/1 -> Detect Increase/1
  Detect Increase1/1 -> 2dbl1/1
  Switch/1 -> state/1, Unit Delay/1
  DSBL/1 -> Detect Increase1/1
  OR/1 -> Switch/2
  Detect Increase/1 -> 2dbl/1
  Unit Delay/1 -> Switch/3
  disable/1 -> Switch1/1
  enable/1 -> Switch1/3
  Switch1/1 -> Switch/1
  2dbl1/1 -> Switch1/2, OR/2
  2dbl/1 -> OR/1

== system BugE_v0_40_MAS_loads_opt/Master Controller/Signal Buffer/(0 device OFF // 1 ON)4 ==
  EN : Inport
  DSBL : Inport  Port=2
  2dbl : DataTypeConversion  OutDataTypeStr=double
  2dbl1 : DataTypeConversion  OutDataTypeStr=double
  Detect Increase : simulink/Logic and Bit Operations/Detect Increase  vinit=0.0  InputProcessing=Inherited  OutDataTypeStr=boolean
  Detect Increase1 : simulink/Logic and Bit Operations/Detect Increase  vinit=0.0  InputProcessing=Inherited  OutDataTypeStr=boolean
  OR : Sum
  Switch : Switch  Criteria=u2 > Threshold
  Switch1 : Switch  Criteria=u2 > Threshold
  Unit Delay : UnitDelay  SampleTime=sample_time
  disable : Constant  Value=0  OutDataTypeStr=boolean  SampleTime=sample_time
  enable : Constant  OutDataTypeStr=boolean  SampleTime=sample_time
  state : Outport
  wires:
  EN/1 -> Detect Increase/1
  Detect Increase1/1 -> 2dbl1/1
  Switch/1 -> state/1, Unit Delay/1
  DSBL/1 -> Detect Increase1/1
  OR/1 -> Switch/2
  Detect Increase/1 -> 2dbl/1
  Unit Delay/1 -> Switch/3
  disable/1 -> Switch1/1
  enable/1 -> Switch1/3
  Switch1/1 -> Switch/1
  2dbl1/1 -> Switch1/2, OR/2
  2dbl/1 -> OR/1

== system BugE_v0_40_MAS_loads_opt/Master Controller/Signal Buffer/(0 device OFF // 1 ON)5 ==
  EN : Inport
  DSBL : Inport  Port=2
  2dbl : DataTypeConversion  OutDataTypeStr=double
  2dbl1 : DataTypeConversion  OutDataTypeStr=double
  Detect Increase : simulink/Logic and Bit Operations/Detect Increase  vinit=0.0  InputProcessing=Inherited  OutDataTypeStr=boolean
  Detect Increase1 : simulink/Logic and Bit Operations/Detect Increase  vinit=0.0  InputProcessing=Inherited  OutDataTypeStr=boolean
  OR : Sum
  Switch : Switch  Criteria=u2 > Threshold
  Switch1 : Switch  Criteria=u2 > Threshold
  Unit Delay : UnitDelay  SampleTime=sample_time
  disable : Constant  Value=0  OutDataTypeStr=boolean  SampleTime=sample_time
  enable : Constant  OutDataTypeStr=boolean  SampleTime=sample_time
  state : Outport
  wires:
  EN/1 -> Detect Increase/1
  Detect Increase1/1 -> 2dbl1/1
  Switch/1 -> state/1, Unit Delay/1
  DSBL/1 -> Detect Increase1/1
  OR/1 -> Switch/2
  Detect Increase/1 -> 2dbl/1
  Unit Delay/1 -> Switch/3
  disable/1 -> Switch1/1
  enable/1 -> Switch1/3
  Switch1/1 -> Switch/1
  2dbl1/1 -> Switch1/2, OR/2
  2dbl/1 -> OR/1

== system BugE_v0_40_MAS_loads_opt/Master Controller/Signal Buffer/(0 device OFF // 1 ON)6 ==
  EN : Inport
  DSBL : Inport  Port=2
  2dbl : DataTypeConversion  OutDataTypeStr=double
  2dbl1 : DataTypeConversion  OutDataTypeStr=double
  Detect Increase : simulink/Logic and Bit Operations/Detect Increase  vinit=0.0  InputProcessing=Inherited  OutDataTypeStr=boolean
  Detect Increase1 : simulink/Logic and Bit Operations/Detect Increase  vinit=0.0  InputProcessing=Inherited  OutDataTypeStr=boolean
  OR : Sum
  Switch : Switch  Criteria=u2 > Threshold
  Switch1 : Switch  Criteria=u2 > Threshold
  Unit Delay : UnitDelay  SampleTime=sample_time
  disable : Constant  Value=0  OutDataTypeStr=boolean  SampleTime=sample_time
  enable : Constant  OutDataTypeStr=boolean  SampleTime=sample_time
  state : Outport
  wires:
  EN/1 -> Detect Increase/1
  Detect Increase1/1 -> 2dbl1/1
  Switch/1 -> state/1, Unit Delay/1
  DSBL/1 -> Detect Increase1/1
  OR/1 -> Switch/2
  Detect Increase/1 -> 2dbl/1
  Unit Delay/1 -> Switch/3
  disable/1 -> Switch1/1
  enable/1 -> Switch1/3
  Switch1/1 -> Switch/1
  2dbl1/1 -> Switch1/2, OR/2
  2dbl/1 -> OR/1

== system BugE_v0_40_MAS_loads_opt/Master Controller/Signal Buffer/(0 device OFF // 1 ON)7 ==
  EN : Inport
  DSBL : Inport  Port=2
  2dbl : DataTypeConversion  OutDataTypeStr=double
  2dbl1 : DataTypeConversion  OutDataTypeStr=double
  Detect Increase : simulink/Logic and Bit Operations/Detect Increase  vinit=0.0  InputProcessing=Inherited  OutDataTypeStr=boolean
  Detect Increase1 : simulink/Logic and Bit Operations/Detect Increase  vinit=0.0  InputProcessing=Inherited  OutDataTypeStr=boolean
  OR : Sum
  Switch : Switch  Criteria=u2 > Threshold
  Switch1 : Switch  Criteria=u2 > Threshold
  Unit Delay : UnitDelay  SampleTime=sample_time
  disable : Constant  Value=0  OutDataTypeStr=boolean  SampleTime=sample_time
  enable : Constant  OutDataTypeStr=boolean  SampleTime=sample_time
  state : Outport
  wires:
  EN/1 -> Detect Increase/1
  Detect Increase1/1 -> 2dbl1/1
  Switch/1 -> state/1, Unit Delay/1
  DSBL/1 -> Detect Increase1/1
  OR/1 -> Switch/2
  Detect Increase/1 -> 2dbl/1
  Unit Delay/1 -> Switch/3
  disable/1 -> Switch1/1
  enable/1 -> Switch1/3
  Switch1/1 -> Switch/1
  2dbl1/1 -> Switch1/2, OR/2
  2dbl/1 -> OR/1

== system BugE_v0_40_MAS_loads_opt/Master Controller/Signal Buffer/(0 device OFF // 1 ON)8 ==
  EN : Inport
  DSBL : Inport  Port=2
  2dbl : DataTypeConversion  OutDataTypeStr=double
  2dbl1 : DataTypeConversion  OutDataTypeStr=double
  Detect Increase : simulink/Logic and Bit Operations/Detect Increase  vinit=0.0  InputProcessing=Inherited  OutDataTypeStr=boolean
  Detect Increase1 : simulink/Logic and Bit Operations/Detect Increase  vinit=0.0  InputProcessing=Inherited  OutDataTypeStr=boolean
  OR : Sum
  Switch : Switch  Criteria=u2 > Threshold
  Switch1 : Switch  Criteria=u2 > Threshold
  Unit Delay : UnitDelay  SampleTime=sample_time
  disable : Constant  Value=0  OutDataTypeStr=boolean  SampleTime=sample_time
  enable : Constant  OutDataTypeStr=boolean  SampleTime=sample_time
  state : Outport
  wires:
  EN/1 -> Detect Increase/1
  Detect Increase1/1 -> 2dbl1/1
  Switch/1 -> state/1, Unit Delay/1
  DSBL/1 -> Detect Increase1/1
  OR/1 -> Switch/2
  Detect Increase/1 -> 2dbl/1
  Unit Delay/1 -> Switch/3
  disable/1 -> Switch1/1
  enable/1 -> Switch1/3
  Switch1/1 -> Switch/1
  2dbl1/1 -> Switch1/2, OR/2
  2dbl/1 -> OR/1

== system BugE_v0_40_MAS_loads_opt/Master Controller/Signal Buffer/(0 device OFF // 1 ON)9 ==
  EN : Inport
  DSBL : Inport  Port=2
  2dbl : DataTypeConversion  OutDataTypeStr=double
  2dbl1 : DataTypeConversion  OutDataTypeStr=double
  Detect Increase : simulink/Logic and Bit Operations/Detect Increase  vinit=0.0  InputProcessing=Inherited  OutDataTypeStr=boolean
  Detect Increase1 : simulink/Logic and Bit Operations/Detect Increase  vinit=0.0  InputProcessing=Inherited  OutDataTypeStr=boolean
  OR : Sum
  Switch : Switch  Criteria=u2 > Threshold
  Switch1 : Switch  Criteria=u2 > Threshold
  Unit Delay : UnitDelay  SampleTime=sample_time
  disable : Constant  Value=0  OutDataTypeStr=boolean  SampleTime=sample_time
  enable : Constant  OutDataTypeStr=boolean  SampleTime=sample_time
  state : Outport
  wires:
  EN/1 -> Detect Increase/1
  Detect Increase1/1 -> 2dbl1/1
  Switch/1 -> state/1, Unit Delay/1
  DSBL/1 -> Detect Increase1/1
  OR/1 -> Switch/2
  Detect Increase/1 -> 2dbl/1
  Unit Delay/1 -> Switch/3
  disable/1 -> Switch1/1
  enable/1 -> Switch1/3
  Switch1/1 -> Switch/1
  2dbl1/1 -> Switch1/2, OR/2
  2dbl/1 -> OR/1

== system BugE_v0_40_MAS_loads_opt/Master Controller/Signal Buffer/RLYs_and_12V_bus ==
  Bus Creator : BusCreator  Inputs=12
  Bus Selector : BusSelector  OutputSignals=RLY_MB_DSBL,RLY_SB_DSBL,RLY_EDLC_DSBL,RLY_AUX_DSBL,RLY_DRV_DSBL,DDC_DSBL
  Bus Selector1 : BusSelector  OutputSignals=RLY_MB_EN,RLY_SB_EN,RLY_EDLC_EN,RLY_AUX_EN,DDC_EN
  Bus Selector2 : BusSelector  OutputSignals=RLY_MB_EN,RLY_SB_EN,RLY_MB_DSBL,RLY_SB_DSBL,RLY_DRV_DSBL
  Bus Selector3 : BusSelector  OutputSignals=RLY_MB_EN,RLY_SB_EN,RLY_MB_DSBL,RLY_SB_DSBL,RLY_DRV_EN
  Gain{,1..6} (7 alike) : Gain  OutDataTypeStr=double
  OR10 : Sum  Inputs=+++  AccumDataTypeStr=double  OutDataTypeStr=double
  OR12 : Sum  OutDataTypeStr=double
  OR7 : Sum  Inputs=+++  OutDataTypeStr=double
  OR8 : Sum  Inputs=+++  OutDataTypeStr=double
  OR9 : Sum  Inputs=+++  OutDataTypeStr=double
  Out1 : Outport
  wires:
  Bus Creator/1 -> Out1/1
  OR10/1 -> Bus Creator/4  "RLY_SB_EN"
  Bus Selector2/2 -> OR10/2  "<RLY_SB_EN>"
  Bus Selector2/5 -> OR12/2  "<RLY_DRV_DSBL>"
  Bus Selector/5 -> OR12/1  "<RLY_DRV_DSBL>"
  OR7/1 -> Bus Creator/1  "RLY_MB_DSBL"
  [RLYs_and_12V_bus3] -> Bus Selector2/1
  Gain5/1 -> Bus Creator/5  "RLY_AUX_DSBL"
  Bus Selector/1 -> OR7/1  "<RLY_MB_DSBL>"
  Bus Selector1/1 -> OR9/1  "<RLY_MB_EN>"
  Gain6/1 -> Bus Creator/7  "RLY_DRV_EN"
  OR9/1 -> Bus Creator/3  "RLY_MB_EN"
  Bus Selector3/2 -> OR10/3  "<RLY_SB_EN>"
  Bus Selector2/4 -> OR8/2  "<RLY_SB_DSBL>"
  Bus Selector1/4 -> Gain3/1  "<RLY_AUX_EN>"
  Bus Selector3/3 -> OR7/3  "<RLY_MB_DSBL>"
  [RLYs_and_12V_bus2] -> Bus Selector1/1
  Bus Selector/4 -> Gain5/1  "<RLY_AUX_DSBL>"
  Bus Selector2/3 -> OR7/2  "<RLY_MB_DSBL>"
  Bus Selector3/4 -> OR8/3  "<RLY_SB_DSBL>"
  Bus Selector3/5 -> Gain6/1  "<RLY_DRV_EN>"
  OR12/1 -> Bus Creator/6  "RLY_DRV_DSBL"
  Bus Selector/6 -> Gain1/1  "<DDC_DSBL>"
  Bus Selector2/1 -> OR9/2  "<RLY_MB_EN>"
  OR8/1 -> Bus Creator/2  "RLY_SB_DSBL"
  Bus Selector1/5 -> Gain4/1  "<DDC_EN>"
  [RLYs_and_12V_bus4] -> Bus Selector3/1
  Bus Selector3/1 -> OR9/3  "<RLY_MB_EN>"
  Bus Selector1/2 -> OR10/1  "<RLY_SB_EN>"
  Bus Selector/3 -> Gain/1  "<RLY_EDLC_DSBL>"
  Bus Selector1/3 -> Gain2/1  "<RLY_EDLC_EN>"
  Bus Selector/2 -> OR8/1  "<RLY_SB_DSBL>"
  [RLYs_and_12V_bus] -> Bus Selector/1
  Gain/1 -> Bus Creator/8  "RLY_EDLC_DSBL"
  Gain1/1 -> Bus Creator/9  "DDC_DSBL"
  Gain2/1 -> Bus Creator/10  "RLY_EDLC_EN"
  Gain3/1 -> Bus Creator/11  "RLY_AUX_EN"
  Gain4/1 -> Bus Creator/12  "DDC_EN"
